simulink model "jwgcqp"  (Simulink 6.0)
settings: Solver=ode23  StartTime=0.0  StopTime=7  FixedStep=0.001  MaxStep=0.003  RelTol=1e-3
InitFcn:
  | jwgcp()
values from neighbouring files (symbols this model uses):
  A = [           0                   1 0             0;     (M+m)*m*g*l/((M+m)*I+M*m*l^2) 0 0 m*l*b/((M+m)*I+M*m*l^2);               0                   0 0             1;      -m^2*l^2*g/((M+m)*I+M*m*l^2) 0 0 -(I+m*l^2)*b/((M+m)*I+M*m*l^2)]    [pendulum.m]    (also in tracker.m = [0 1 0 0;51.58 0 0 0.5263;0 0 0 1;-7.737 0 0 -0.1789])
  A11 = A1(1:q,1:q)    [jwgcl.m]    (also in jwgcp.m)
  A12 = A1(1:q,q+1:4)    [jwgcl.m]    (also in jwgcp.m)
  A21 = A1(q+1:4,1:q)    [jwgcl.m]    (also in jwgcp.m)
  A22 = A1(q+1:4,q+1:4)    [jwgcl.m]    (also in jwgcp.m)
  B = [0;-m*l/(((M+m)*I+M*m*l^2));0;(I+m*l^2)/((M+m)*I+M*m*l^2)]    [pendulum.m]    (also in tracker.m = [0;-5.263;0;1.789])
  B11 = B1(1:q,:)    [jwgcl.m]    (also in jwgcp.m)
  B12 = B1(q+1:4,:)    [jwgcl.m]    (also in jwgcp.m)
  C = [0 0 1 0;1 0 0 0]    [pendulum.m]    (also in tracker.m = [0 0 1 0])
  Ks = lqr(A,B,Q,R)    [jwgcl.m]    (also in jwgcp.m = [0 0 0 1]*inv(Qc)*PP; pendulum.m = lqr(A,B,QQ,RR))
  L = K'    [jwgcl.m]    (also in jwgcp.m)
  Q1 = Q(:,1:q)    [jwgcl.m]    (also in jwgcp.m)
  Q2 = Q(:,q+1:rank(Q))    [jwgcl.m]    (also in jwgcp.m)
settings Model: LastModifiedBy=Administrator
settings DataIOCC: SignalLoggingName=sigsOut
settings DebuggingCC: SolverPrmCheckMsg=none
settings HardwareCC: TargetUnknown=on

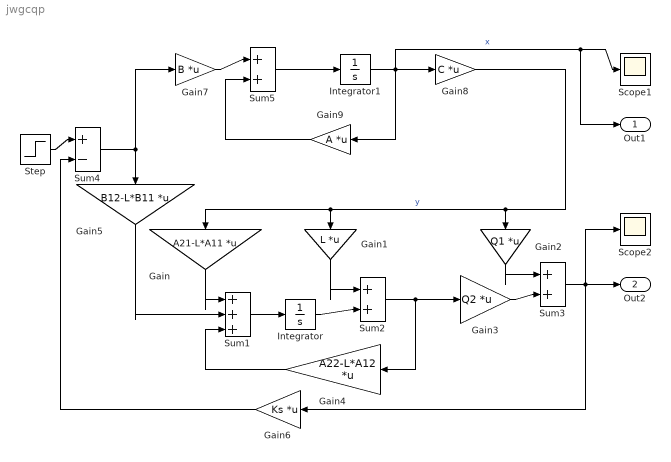
== system jwgcqp ==
  Gain : Gain  Orientation=down  Gain=A21-L*A11  Multiplication=Matrix(K*u)  SaturateOnIntegerOverflow=on
  Gain1 : Gain  Orientation=down  Gain=L  Multiplication=Matrix(K*u)  SaturateOnIntegerOverflow=on
  Gain2 : Gain  Orientation=down  Gain=Q1  Multiplication=Matrix(K*u)  SaturateOnIntegerOverflow=on
  Gain3 : Gain  Gain=Q2  Multiplication=Matrix(K*u)  SaturateOnIntegerOverflow=on
  Gain4 : Gain  Orientation=left  Gain=A22-L*A12  Multiplication=Matrix(K*u)  SaturateOnIntegerOverflow=on
  Gain5 : Gain  Orientation=down  Gain=B12-L*B11  Multiplication=Matrix(K*u)  SaturateOnIntegerOverflow=on
  Gain6 : Gain  Orientation=left  Gain=Ks  Multiplication=Matrix(K*u)  SaturateOnIntegerOverflow=on
  Gain7 : Gain  Gain=B  Multiplication=Matrix(K*u)  SaturateOnIntegerOverflow=on
  Gain8 : Gain  Gain=C  Multiplication=Matrix(K*u)  SaturateOnIntegerOverflow=on
  Gain9 : Gain  Orientation=left  Gain=A  Multiplication=Matrix(K*u)  SaturateOnIntegerOverflow=on
  Integrator : Integrator
  Integrator1 : Integrator
  Scope1 : Scope
      settings: TimeRange=10  SaveName=ScopeData4
  Scope2 : Scope
  Step : Step  Time=0  After=0.2  SampleTime=0  VectorParams1D=off
  Sum1 : Sum  Inputs=|+++  SaturateOnIntegerOverflow=on
  Sum2 : Sum  Inputs=|++  SaturateOnIntegerOverflow=on
  Sum3 : Sum  Inputs=|++  SaturateOnIntegerOverflow=on
  Sum4 : Sum  Inputs=|+-  SaturateOnIntegerOverflow=on
  Sum5 : Sum  Inputs=|++  SaturateOnIntegerOverflow=on
  Out1 : Outport
  Out2 : Outport  Port=2
  wires:
  Gain/1 -> Sum1/1
  Sum1/1 -> Integrator/1
  Gain1/1 -> Sum2/1
  Integrator/1 -> Sum2/2
  Sum2/1 -> Gain3/1, Gain4/1
  Gain2/1 -> Sum3/1
  Gain3/1 -> Sum3/2
  Sum3/1 -> Gain6/1, Out2/1, Scope2/1
  Gain4/1 -> Sum1/3
  Gain5/1 -> Sum1/2
  Sum4/1 -> Gain5/1, Gain7/1
  Step/1 -> Sum4/1
  Gain6/1 -> Sum4/2
  Gain7/1 -> Sum5/1
  Sum5/1 -> Integrator1/1
  Integrator1/1 -> Gain8/1, Gain9/1, Out1/1, Scope1/1  "x"
  Gain8/1 -> Gain/1, Gain1/1, Gain2/1  "y"
  Gain9/1 -> Sum5/2
